simulink model "ControlledRectifier"  (R2025a)
settings: Solver=FixedStepDiscrete  StartTime=0.0  StopTime=1  FixedStep=1e-0.5  RelTol=1e-3
libraries: spsThyristorLib x4, spsMeanLib x2, eeRmsMeasurement x2, spsVoltageMeasurementLib x2, spsACVoltageSourceLib x1, spsCurrentMeasurementLib x1, spsSeriesRLCBranchLib x1, spspowerguiLib x1
settings Model: Creator=Jaime  LastModifiedBy=Jaime

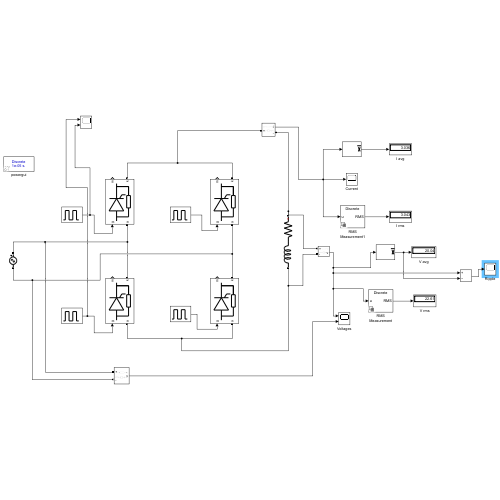
[thumbnail: Simulink's stored preview of the top-level diagram]
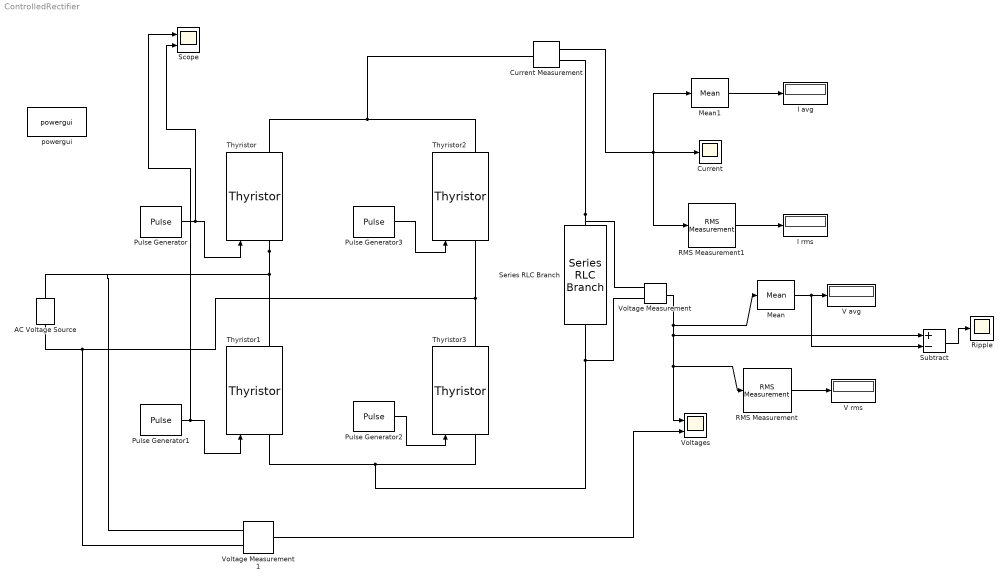
== system ControlledRectifier ==
  AC Voltage Source : spsACVoltageSourceLib/AC Voltage Source  Amplitude=34  Phase=0  Frequency=60  SampleTime=0  Measurements=None  BusType=swing  Pref=10e3  Qref=0  Qmin=-inf  Qmax=+inf
  Current : Scope
      settings: TimeSpan=1/25  TimeUnits=Metric (based on Time Span)  ActiveDisplayYMinimum=-1.1982988296301262  ActiveDisplayYMaximum=4.7608828371183964
  Current Measurement : spsCurrentMeasurementLib/Current Measurement  PhasorSimulation=off  OutputType=Complex  PSBequivalent=0
  I avg : Display
  I rms : Display
  Mean : spsMeanLib/Mean  Freq=60  Vinit=0  Ts=1/(60*200)
  Mean1 : spsMeanLib/Mean  Freq=60  Vinit=0  Ts=1/(60*200)
  Pulse Generator : DiscretePulseGenerator  PulseType=Time based  Period=1/60  PulseWidth=5  PhaseDelay=(1)*0.016667/360
  Pulse Generator1 : DiscretePulseGenerator  PulseType=Time based  Period=1/60  PulseWidth=5  PhaseDelay=(0+180)*0.016667/360
  Pulse Generator2 : DiscretePulseGenerator  PulseType=Time based  Period=1/60  PulseWidth=5  PhaseDelay=1*0.0166673/360
  Pulse Generator3 : DiscretePulseGenerator  PulseType=Time based  Period=1/60  PulseWidth=5  PhaseDelay=(0+180)*0.016667/360
  RMS Measurement : eeRmsMeasurement/RMS Measurement  LabelModeActiveChoice=Total  F=60  SpecifyHarmonics=off  K=[0 1 2]  Ts=1/(60*200)
      settings: LibrarySourceBlock=|
      | ee_sl_lib/Measurements/RMS
      | Measurement
  RMS Measurement1 : eeRmsMeasurement/RMS Measurement  LabelModeActiveChoice=Total  F=60  SpecifyHarmonics=off  K=[0 1 2]  Ts=1/(60*200)
      settings: LibrarySourceBlock=|
      | ee_sl_lib/Measurements/RMS
      | Measurement
  Ripple : Scope
      settings: ActiveDisplayYMinimum=-35.439609961313955  ActiveDisplayYMaximum=51.879193991056049  DataLoggingVariableName=ScopeData3
  Scope : Scope  NumInputPorts=2
      settings: ActiveDisplayYMinimum=-0.12499999999999997  ActiveDisplayYMaximum=1.125  DataLoggingVariableName=ScopeData2
  Series RLC Branch : spsSeriesRLCBranchLib/Series RLC Branch  LConnTagsString=__new0  RConnTagsString=__new0  BranchType=RL  Resistance=6.6  Inductance=.065  SetiL0=off  InitialCurrent=0  Capacitance=0  Setx0=off  InitialVoltage=0  Measurements=Branch voltage and current
  Subtract : Sum  Inputs=+-
  Thyristor{,1..3} (4 alike) : spsThyristorLib/Thyristor  Ron=0.001  Lon=0  Vf=0.8  IC=0  Rs=500  Cs=250e-9  Measurements=on
  V avg : Display
  V rms : Display
  Voltage Measurement : spsVoltageMeasurementLib/Voltage Measurement  PhasorSimulation=off  OutputType=Complex  PSBequivalent=0
  Voltage Measurement1 : spsVoltageMeasurementLib/Voltage Measurement  PhasorSimulation=off  OutputType=Complex  PSBequivalent=0
  Voltages : Scope  NumInputPorts=2
      settings: ActiveDisplayYMinimum=-16.746799508783727  ActiveDisplayYMaximum=51.904128416200393
  powergui : spspowerguiLib/powergui  Priority=1  SimulationMode=Discrete  SampleTime=1e-5  frequency=60  Iterations=50  frequencyindice=60  Pbase=100e6  ErrMax=1e-4  UnitsV=kV  UnitsW=MW  buscounter=0  FunctionMessages=off  echomessages=off  EnableUseOfTLC=off  CurrentSourceSwitches=off  DisableSnubberDevices=off  DisableRonSwitches=off  DisableVfSwitches=off  DisplayEquations=off  AutomaticDiscreteSolvers=off  SolverType=Tustin/Backward Euler (TBE)  Interpol=off  ExternalGateDelay=off  methode=off  Ts=100  x0status=blocks  SPID=on  SwTol=0  HookPort=off  NonlinearTolerance=1e-4  nMaxIteration=100  ContinueOnMaxIteration=off  RestoreLinks=warning  ResistiveCurrentMeasurement=off  Frange=[0:2:500]  Ylog=off  Xlog=on  ShowGrid=off  save=off  variable=ZData  structure=0  ZoomFFT=off  StartTime=0.0  cycles=1  DisplayStyle=1  fundamental=60  FreqAxis=off  MaxFrequency=1000  frequencyindicesteady=1  RmsSteady=1  display=off
  wires:
  Pulse Generator3/1 -> Thyristor2/1
  Pulse Generator1/1 -> Scope/1, Thyristor1/1
  Pulse Generator2/1 -> Thyristor3/1
  Pulse Generator/1 -> Scope/2, Thyristor/1
  Voltage Measurement/1 -> Subtract/1, Voltages/1, RMS Measurement/1, Mean/1
  Mean/1 -> Subtract/2, V avg/1
  RMS Measurement/1 -> V rms/1
  Voltage Measurement1/1 -> Voltages/2
  Current Measurement/1 -> RMS Measurement1/1, Current/1, Mean1/1
  Mean1/1 -> I avg/1
  RMS Measurement1/1 -> I rms/1
  Subtract/1 -> Ripple/1
  connections:
  Thyristor/LConn1 -- AC Voltage Source/RConn1 -- Voltage Measurement1/LConn1 -- Thyristor1/RConn1
  Thyristor3/RConn1 -- Thyristor2/LConn1 -- AC Voltage Source/LConn1 -- Voltage Measurement1/LConn2
  Thyristor3/LConn1 -- Thyristor1/LConn1 -- Voltage Measurement/LConn2 -- Series RLC Branch/RConn1
  Thyristor/RConn1 -- Current Measurement/LConn1 -- Thyristor2/RConn1
  Current Measurement/RConn1 -- Voltage Measurement/LConn1 -- Series RLC Branch/LConn1
